simulink model "ba_xe"  (R2021b)
settings: Solver=FixedStepAuto  StartTime=0.0  StopTime=15  FixedStep=0.01  RelTol=1e-3
settings Model: Creator=HL_1810  LastModifiedBy=SPKT2021

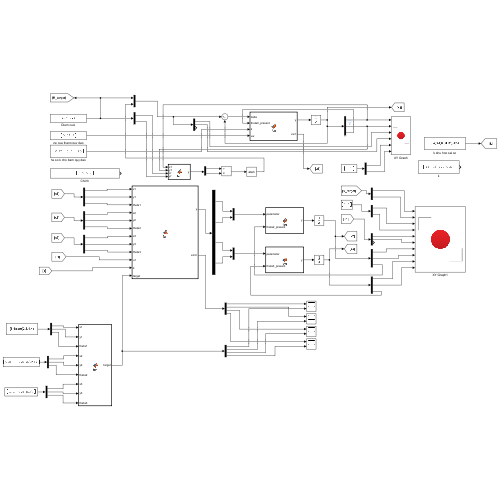
[thumbnail: Simulink's stored preview of the top-level diagram]
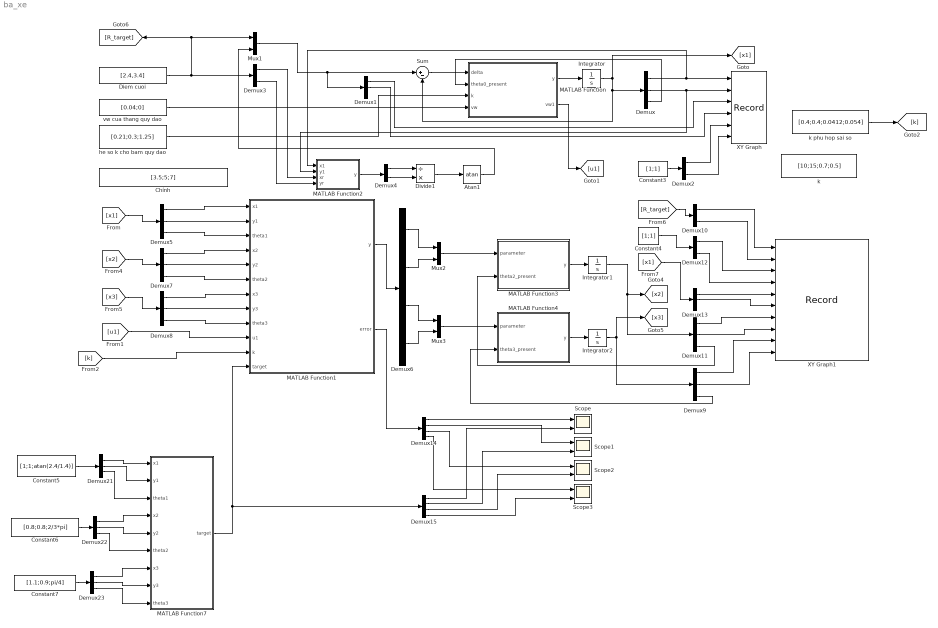
== system ba_xe ==
  Atan1 : Trigonometry  Operator=atan
  Chính : Constant  Value=[3.5;5;7]
  Constant3 : Constant  Value=[1;1]
  Constant4 : Constant  Value=[1;1]
  Constant5 : Constant  Value=[1;1;atan(2.4/1.4)]
  Constant6 : Constant  Value=[0.8;0.8;2/3*pi]
  Constant7 : Constant  Value=[1.1;0.9;pi/4]
  Demux{,1,5,7..9,11,13,21..23} (11 alike) : Demux  Outputs=3
  Demux{2..4,10,12} (5 alike) : Demux  Outputs=2
  Demux14 : Demux
  Demux15 : Demux
  Demux6 : Demux
  Diem cuoi : Constant  Value=[2.4,3.4]
  Divide1 : Product  Inputs=/*
  Integrator : Integrator  InitialCondition=[1;1;atan(2.4/1.4)]
  Integrator1 : Integrator  InitialCondition=[0.8;0.8;2/3*pi]
  Integrator2 : Integrator  InitialCondition=[1.1;0.9;pi/4]
  MATLAB Function : MATLAB Function  TreatAsAtomicUnit=on
  MATLAB Function1 : MATLAB Function  TreatAsAtomicUnit=on
  MATLAB Function2 : MATLAB Function  TreatAsAtomicUnit=on
  MATLAB Function3 : MATLAB Function  TreatAsAtomicUnit=on
  MATLAB Function4 : MATLAB Function  TreatAsAtomicUnit=on
  MATLAB Function7 : MATLAB Function  TreatAsAtomicUnit=on
  Mux1 : Mux  Inputs=2
  Mux2 : Mux  Inputs=2
  Mux3 : Mux  Inputs=2
  Scope{,1..3} (4 alike) : Scope  NumInputPorts=2
  Sum : Sum  Inputs=|+-
  XY Graph : Record  FileSettingsInternal="{\"entries\":[{\"content\":{\"excelSettings\":{\"content\":{},\"type\":\"Streamout.ExcelSettings\"}},\"type\":\"Streamout.FileSettingStorage\",\"uuid\":\"913d583a-c7ca-4ae4-b2df-6f825b279ffb\"}],\"packageUris\":[\"http://schema.mathworks.com/mf0/streamout_blocks/R2020a\"],\"version\":\"1.0\"}"  Layout=[1 1]  SignalsInternal="{\"entries\":[{\"content\":{\"signals\":[{\"content\":{\"blockPath\":[\"ba_xe/XY Graph\"],\"channel\":[],\"dimensions\":[1],\"domain\":\"ba_xe/XY Graph\",\"lineColor\":\"#edb120\",\"plots\":[1],\"port\":1,\"sid\":[\"\"],\"signalID\":1417,\"signalName\":\"Demux:1\"},\"type\":\"RecordBlkView.Signal\",\"uuid\":\"835e361d-6005-4225-8b89-f50d614e2cb5\"},{\"content\":{\"blockPath\":[\"ba_xe/XY Graph\"],\"channel\":[],\"dimensions\":[1],\"domain\":\"ba_xe/XY Graph\",\"lineColor\":\"#7e2f8e\",\"plots\":[1],\"port\":2,\"sid\":[\"\"],\"signalID\":1421,\"signalName\":\"Demux:2\"},\"type\":\"RecordBlkView.Signal\",\"uuid\":\"a13c7c6d-6f06-4c1b-93d2-bab6fcd1b877\"},{\"content\":{\"blockPath\":[\"ba_xe/XY Graph\"],\"channel\":[],\"dimensions\":[1],\"domain\":\"ba_xe/XY Graph\",\"lineColor\":\"#77ac30\",\"plots\":[1],\"port\":3,\"sid\":[\"\"],\"signalID\":1449,\"signalName\":\"Demux1:1\"},\"type\":\"RecordBlkView.Signal\",\"uuid\":\"27da4c3b-8ded-4eca-b8ac-f35d4519574c\"},{\"content\":{\"blockPath\":[\"ba_xe/XY Graph\"],\"channel\":[],\"dimensions\":[1],\"domain\":\"ba_xe/XY Graph\",\"lineColor\":\"#4dbeee\",\"plots\":[1],\"port\":4,\"sid\":[\"\"],\"signalID\":1453,\"signalName\":\"Demux1:2\"},\"type\":\"RecordBlkView.Signal\",\"uuid\":\"ab7d5066-e5c7-44ec-8f84-9db4c2ffea56\"},{\"content\":{\"blockPath\":[\"ba_xe/XY Graph\"],\"channel\":[],\"dimensions\":[1],\"domain\":\"ba_xe/XY Graph\",\"lineColor\":\"#a2142f\",\"plots\":[1],\"port\":5,\"sid\":[\"\"],\"signalID\":1457,\"signalName\":\"Demux2:1\"},\"type\":\"RecordBlkView.Signal\",\"uuid\":\"eb6a5c8b-c41f-4211-8d60-bb920ce87cb9\"},{\"content\":{\"blockPath\":[\"ba_xe/XY Graph\"],\"channel\":[],\"dimensions\":[1],\"domain\":\"ba_xe/XY Graph\",\"lineColor\":\"#139fff\",\"plots\":[1],\"port\":6,\"sid\":[\"\"],\"signalID\":1461,\"signalName\":\"Demux2:2\"},\"type\":\"RecordBlkView.Signal\",\"uuid\":\"f81c33f0-96ee-49dd-8d04-247ed2e1b504\"}]},\"type\":\"RecordBlkView.InputSignals\",\"uuid\":\"6fb8fdba-83d3-4a1b-84ed-ed0fa2a9030c\"}],\"packageUris\":[\"http://schema.mathworks.com/mf0/streamout_blocks/R2020a\"],\"version\":\"1.0\"}"  VisualizationBindings="{\"xyplotplugin\":{\"info\":[{\"series\":[{\"bindingParametersList\":[{\"parameter\":\"X-Axis\",\"signalID\":1449,\"signalName\":\"Demux1:1\"},{\"parameter\":\"Y-Axis\",\"signalID\":1453,\"signalName\":\"Demux1:2\"}],\"seriesID\":6565},{\"bindingParametersList\":[{\"parameter\":\"X-Axis\",\"signalID\":1417,\"signalName\":\"Demux:1\"},{\"parameter\":\"Y-Axis\",\"signalID\":1421,\"signalName\":\"Demux:2\"}],\"seriesID\":57224},{\"bindingParametersList\":[{\"parameter\":\"X-Axis\",\"signalID\":1457,\"signalName\":\"Demux2:1\"},{\"parameter\":\"Y-Axis\",\"signalID\":1461,\"signalName\":\"Demux2:2\"}],\"seriesID\":46579}],\"subplotID\":1},{\"series\":[],\"subplotID\":2}]}}"  CompatibilityTag=XY
  XY Graph1 : Record  FileSettingsInternal="{\"entries\":[{\"content\":{\"excelSettings\":{\"content\":{},\"type\":\"Streamout.ExcelSettings\"}},\"type\":\"Streamout.FileSettingStorage\",\"uuid\":\"9180f49e-0466-4a03-b380-b3340658523c\"}],\"packageUris\":[\"http://schema.mathworks.com/mf0/streamout_blocks/R2020a\"],\"version\":\"1.0\"}"  Layout=[1 1]  SignalsInternal="{\"entries\":[{\"content\":{\"signals\":[{\"content\":{\"blockPath\":[\"ba_xe/XY Graph1\"],\"channel\":[],\"dimensions\":[1],\"domain\":\"ba_xe/XY Graph1\",\"lineColor\":\"#64d413\",\"plots\":[1],\"port\":5,\"sid\":[\"\"],\"signalID\":1425,\"signalName\":\"Demux13:1\"},\"type\":\"RecordBlkView.Signal\",\"uuid\":\"40623cd3-fd37-4be6-82f0-8d19e25bf14b\"},{\"content\":{\"blockPath\":[\"ba_xe/XY Graph1\"],\"channel\":[],\"dimensions\":[1],\"domain\":\"ba_xe/XY Graph1\",\"lineColor\":\"#ff13a6\",\"plots\":[1],\"port\":6,\"sid\":[\"\"],\"signalID\":1429,\"signalName\":\"Demux13:2\"},\"type\":\"RecordBlkView.Signal\",\"uuid\":\"b040d25c-6858-404a-8bcf-27572d0b4264\"},{\"content\":{\"blockPath\":[\"ba_xe/XY Graph1\"],\"channel\":[],\"dimensions\":[1,1],\"domain\":\"ba_xe/XY Graph1\",\"lineColor\":\"#fe330a\",\"plots\":[1],\"port\":7,\"sid\":[\"\"],\"signalID\":1433,\"signalName\":\"Demux11:1\"},\"type\":\"RecordBlkView.Signal\",\"uuid\":\"01219603-0774-4d1b-85fd-df1bd27ad9f9\"},{\"content\":{\"blockPath\":[\"ba_xe/XY Graph1\"],\"channel\":[],\"dimensions\":[1,1],\"domain\":\"ba_xe/XY Graph1\",\"lineColor\":\"#22b573\",\"plots\":[1],\"port\":8,\"sid\":[\"\"],\"signalID\":1437,\"signalName\":\"Demux11:2\"},\"type\":\"RecordBlkView.Signal\",\"uuid\":\"0880b329-3556-49db-af49-48faf31e40ef\"},{\"content\":{\"blockPath\":[\"ba_xe/XY Graph1\"],\"channel\":[],\"dimensions\":[1,1],\"domain\":\"ba_xe/XY Graph1\",\"lineColor\":\"#a2142f\",\"plots\":[1],\"port\":9,\"sid\":[\"\"],\"signalID\":1441,\"signalName\":\"Demux9:1\"},\"type\":\"RecordBlkView.Signal\",\"uuid\":\"70a5cc00-347b-48cf-802a-643db1fc47df\"},{\"content\":{\"blockPath\":[\"ba_xe/XY Graph1\"],\"channel\":[],\"dimensions\":[1,1],\"domain\":\"ba_xe/XY Graph1\",\"lineColor\":\"#139fff\",\"plots\":[1],\"port\":10,\"sid\":[\"\"],\"signalID\":1445,\"signalName\":\"Demux9:2\"},\"type\":\"RecordBlkView.Signal\",\"uuid\":\"d5dcc1ee-4cc6-40ee-997e-a3217fc7e3ef\"},{\"content\":{\"blockPath\":[\"ba_xe/XY Graph1\"],\"channel\":[],\"dimensions\":[1],\"domain\":\"ba_xe/XY Graph1\",\"lineColor\":\"#a2142f\",\"plots\":[1],\"port\":1,\"sid\":[\"\"],\"signalID\":1465,\"signalName\":\"Demux10:1\"},\"type\":\"RecordBlkView.Signal\",\"uuid\":\"d015556c-0021-4f36-8523-1ea12413921d\"},{\"content\":{\"blockPath\":[\"ba_xe/XY Graph1\"],\"channel\":[],\"dimensions\":[1],\"domain\":\"ba_xe/XY Graph1\",\"lineColor\":\"#139fff\",\"plots\":[1],\"port\":2,\"sid\":[\"\"],\"signalID\":1469,\"signalName\":\"Demux10:2\"},\"type\":\"RecordBlkView.Signal\",\"uuid\":\"5dec3d70-aef2-47e4-8f63-af19e4fd09ad\"},{\"content\":{\"blockPath\":[\"ba_xe/XY Graph1\"],\"channel\":[],\"dimensions\":[1],\"domain\":\"ba_xe/XY Graph1\",\"lineColor\":\"#ff6929\",\"plots\":[1],\"port\":3,\"sid\":[\"\"],\"signalID\":1473,\"signalName\":\"Demux12:1\"},\"type\":\"RecordBlkView.Signal\",\"uuid\":\"90f3538a-7199-4069-b5b5-c1cc89a0668e\"},{\"content\":{\"blockPath\":[\"ba_xe/XY Graph1\"],\"channel\":[],\"dimensions\":[1],\"domain\":\"ba_xe/XY Graph1\",\"lineColor\":\"#b746ff\",\"plots\":[1],\"port\":4,\"sid\":[\"\"],\"signalID\":1477,\"signalName\":\"Demux12:2\"},\"type\":\"RecordBlkView.Signal\",\"uuid\":\"e6ec1e45-6779-4edb-ad73-a0428db076df\"}]},\"type\":\"RecordBlkView.InputSignals\",\"uuid\":\"0dbc682c-6d13-4a69-b4bd-1c5f65b30b30\"}],\"packageUris\":[\"http://schema.mathworks.com/mf0/streamout_blocks/R2020a\"],\"version\":\"1.0\"}"  VisualizationBindings="{\"xyplotplugin\":{\"info\":[{\"series\":[{\"bindingParametersList\":[{\"parameter\":\"X-Axis\",\"signalID\":1441,\"signalName\":\"Demux9:1\"},{\"parameter\":\"Y-Axis\",\"signalID\":1445,\"signalName\":\"Demux9:2\"}],\"seriesID\":12018},{\"bindingParametersList\":[{\"parameter\":\"X-Axis\",\"signalID\":1465,\"signalName\":\"Demux10:1\"},{\"parameter\":\"Y-Axis\",\"signalID\":1469,\"signalName\":\"Demux10:2\"}],\"seriesID\":34676},{\"bindingParametersList\":[{\"parameter\":\"X-Axis\",\"signalID\":1473,\"signalName\":\"Demux12:1\"},{\"parameter\":\"Y-Axis\",\"signalID\":1477,\"signalName\":\"Demux12:2\"}],\"seriesID\":29055},{\"bindingParametersList\":[{\"parameter\":\"X-Axis\",\"signalID\":1433,\"signalName\":\"Demux11:1\"},{\"parameter\":\"Y-Axis\",\"signalID\":1437,\"signalName\":\"Demux11:2\"}],\"seriesID\":28197},{\"bindingParametersList\":[{\"parameter\":\"X-Axis\",\"signalID\":1425,\"signalName\":\"Demux13:1\"},{\"parameter\":\"Y-Axis\",\"signalID\":1429,\"signalName\":\"Demux13:2\"}],\"seriesID\":62140}],\"subplotID\":1},{\"series\":[],\"subplotID\":2},{\"series\":[],\"subplotID\":9},{\"series\":[],\"subplotID\":10}]}}"  CompatibilityTag=XY
  he so k cho bam quy dao : Constant  Value=[0.21;0.3;1.25]
  k : Constant  Value=[10;15;0.7;0.5]
  k phu hop sai so : Constant  Value=[0.4;0.4;0.0412;0.054]
  vw cua thang quy dao : Constant  Value=[0.04;0]
  wires:
  Sum/1 -> MATLAB Function/1(delta)
  he so k cho bam quy dao/1 -> MATLAB Function/3(k)
  Demux2/1 -> XY Graph/5
  Demux/1 -> MATLAB Function2/1(x1), XY Graph/1
  Mux1/1 -> Sum/1, Demux1/1
  Demux3/2 -> MATLAB Function2/4(yr)
  Demux1/1 -> XY Graph/3
  Demux2/2 -> XY Graph/6
  Divide1/1 -> Atan1/1
  vw cua thang quy dao/1 -> MATLAB Function/4(vw)
  Constant3/1 -> Demux2/1
  Diem cuoi/1 -> [R_target], Mux1/1, Demux3/1
  MATLAB Function/1(y) -> Integrator/1
  Atan1/1 -> Mux1/2
  Demux/3 -> MATLAB Function/2(theta0_present)
  MATLAB Function2/1(y) -> Demux4/1
  Integrator/1 -> Sum/2, Demux/1, [x1]
  Demux3/1 -> MATLAB Function2/3(xr)
  Demux1/2 -> XY Graph/4
  Demux/2 -> MATLAB Function2/2(y1), XY Graph/2
  Demux5/1 -> MATLAB Function1/1(x1)
  Mux2/1 -> MATLAB Function3/1(parameter)
  Demux8/2 -> MATLAB Function1/8(y3)
  Demux8/1 -> MATLAB Function1/7(x3)
  Demux9/3 -> MATLAB Function4/2(theta3_present)
  Integrator2/1 -> [x3], Demux9/1
  [x3] -> Demux8/1
  Demux11/3 -> MATLAB Function3/2(theta2_present)
  [u1] -> MATLAB Function1/10(u1)
  MATLAB Function4/1(y) -> Integrator2/1
  Mux3/1 -> MATLAB Function4/1(parameter)
  Demux7/3 -> MATLAB Function1/6(theta2)
  Demux7/2 -> MATLAB Function1/5(y2)
  Demux5/3 -> MATLAB Function1/3(theta1)
  Demux6/3 -> Mux3/1
  Demux6/4 -> Mux3/2
  Demux6/1 -> Mux2/1
  Demux8/3 -> MATLAB Function1/9(theta3)
  Demux5/2 -> MATLAB Function1/2(y1)
  Demux7/1 -> MATLAB Function1/4(x2)
  Integrator1/1 -> Demux11/1, [x2]
  [x2] -> Demux7/1
  Demux6/2 -> Mux2/2
  MATLAB Function3/1(y) -> Integrator1/1
  [x1] -> Demux5/1
  MATLAB Function1/1(y) -> Demux6/1
  [k] -> MATLAB Function1/11(k)
  MATLAB Function/2(vw1) -> [u1]
  [R_target] -> Demux10/1
  Demux10/1 -> XY Graph1/1
  Demux10/2 -> XY Graph1/2
  Constant4/1 -> Demux12/1
  Demux12/1 -> XY Graph1/3
  Demux12/2 -> XY Graph1/4
  [x1] -> Demux13/1
  Demux13/1 -> XY Graph1/5
  Demux13/2 -> XY Graph1/6
  Demux11/1 -> XY Graph1/7
  Demux11/2 -> XY Graph1/8
  Demux9/1 -> XY Graph1/9
  Demux9/2 -> XY Graph1/10
  Demux4/2 -> Divide1/2
  Demux4/1 -> Divide1/1
  MATLAB Function1/2(error) -> Demux14/1
  Demux14/1 -> Scope/1
  Demux15/1 -> Scope/2
  Demux14/2 -> Scope1/1
  Demux15/2 -> Scope1/2
  Demux14/3 -> Scope2/1
  Demux15/3 -> Scope2/2
  Demux14/4 -> Scope3/1
  Demux15/4 -> Scope3/2
  k phu hop sai so/1 -> [k]
  Demux23/2 -> MATLAB Function7/8(y3)
  Demux23/1 -> MATLAB Function7/7(x3)
  Constant5/1 -> Demux21/1
  Demux21/1 -> MATLAB Function7/1(x1)
  Demux23/3 -> MATLAB Function7/9(theta3)
  Demux22/3 -> MATLAB Function7/6(theta2)
  Demux21/2 -> MATLAB Function7/2(y1)
  Constant6/1 -> Demux22/1
  Demux22/1 -> MATLAB Function7/4(x2)
  Demux22/2 -> MATLAB Function7/5(y2)
  Demux21/3 -> MATLAB Function7/3(theta1)
  Constant7/1 -> Demux23/1
  MATLAB Function7/1(target) -> Demux15/1, MATLAB Function1/12(target)

== matlab function ba_xe/MATLAB Function1 ==
  data: x1 input; y output; y1 input; theta1 input; x2 input; y2 input; theta2 input; x3 input; y3 input; theta3 input; u1 input; k input; target input; error output
function [y,error] = fcn(x1,y1,theta1,x2,y2,theta2,x3,y3,theta3,u1,k,target)
%#coegen
d=0.09;

L12_x=x1-x2-d*cos(theta2);
L12_y=y1-y2-d*sin(theta2);
L13_x=x1-x3-d*cos(theta3);
L13_y=y1-y3-d*sin(theta3);
L23_x=x2-x3-d*cos(theta3);
L23_y=y2-y3-d*sin(theta3);

L12=sqrt(L12_x^2+L12_y^2);
L13=sqrt(L13_x^2+L13_y^2);
L23=sqrt(L23_x^2+L23_y^2);

mega12=atan(L12_y/L12_x)-theta1+pi;
mega13=atan(L13_y/L13_x)-theta1+pi;
mega23=atan(L23_y/L23_x)-theta2+pi;

beta12=theta1-theta2;
beta13=theta1-theta3;
beta23=theta2-theta3;

si12=beta12+mega12;
si13=beta13+mega13;
si23=beta23+mega23;

G2=[cos(si12)      d*sin(si12)     0         0;
    -sin(si12)/L12 d*cos(si12)/L12 0         0;
    0              0               cos(si13) d*sin(si13);
    -cos(mega23)   0               cos(si23) d*sin(si23)];

F2=[-cos(mega12)     0;
    sin(mega12)/L12 -1;
    -cos(mega13)     0;
    0                0];
p= [k(1)*(target(1)-L12);
    k(2)*(target(2)-mega12);
    k(3)*(target(3)-L13);
    k(4)*(target(4)-L23)];
e=[L12;
mega12;
L13;
L23];

u=inv(G2)*(p-F2*u1);
error=e;
y = u;

== matlab function ba_xe/MATLAB Function ==
  data: delta input; y output; theta0_present input; k input; vw input; vw1 output
function [y,vw1] = fcn(delta,theta0_present,k,vw)
%#codegen
A=[cos(theta0_present)   sin(theta0_present) 0;
    -sin(theta0_present) cos(theta0_present) 0;
    0                    0                    1];
e=A*delta;
V_c=[vw(1)*cos(e(3))+k(1)*e(1);
    vw(2)+k(2)*vw(1)*e(2)+k(3)*vw(1)*sin(e(3))];
Matrix=[cos(theta0_present) 0;
        sin(theta0_present) 0;
        0                   1];
u=Matrix*V_c;
y = u;
vw1=V_c;

== matlab function ba_xe/MATLAB Function2 ==
  data: x1 input; y output; y1 input; xr input; yr input
function y = fcn(x1,y1,xr,yr)
%#codegen
x_delta=xr-x1;
y_delta=yr-y1;
u=[x_delta;y_delta]
y = u;

== matlab function ba_xe/MATLAB Function3 ==
  data: parameter input; y output; theta2_present input
function y = fcn(parameter,theta2_present)
%#codegen
Matrix=[cos(theta2_present) 0;
        sin(theta2_present) 0;
        0                   1];
u=Matrix*parameter;
y = u;

== matlab function ba_xe/MATLAB Function4 ==
  data: parameter input; y output; theta3_present input
function y = fcn(parameter,theta3_present)
%#codegen
Matrix=[cos(theta3_present) 0;
        sin(theta3_present) 0;
        0                   1];
u=Matrix*parameter;
y = u;

== matlab function ba_xe/MATLAB Function7 ==
  data: x1 input; target output; y1 input; theta1 input; x2 input; y2 input; theta2 input; x3 input; y3 input; theta3 input
function target = fcn(x1,y1,theta1,x2,y2,theta2,x3,y3,theta3)
%#codegen
d=0.09;

L12_x=x1-x2-d*cos(theta2);
L12_y=y1-y2-d*sin(theta2);
L13_x=x1-x3-d*cos(theta3);
L13_y=y1-y3-d*sin(theta3);
L23_x=x2-x3-d*cos(theta3);
L23_y=y2-y3-d*sin(theta3);

L12=sqrt(L12_x^2+L12_y^2);
L13=sqrt(L13_x^2+L13_y^2);
L23=sqrt(L23_x^2+L23_y^2);

mega12=atan(L12_y/L12_x)-theta1+pi;
target=[L12;mega12;L13;L23];
